simulink model "diophantineMPCSimulink"  (R2023b)
settings: Solver=VariableStepAuto  StartTime=0.0  StopTime=Tsim  RelTol=1e-3
undefined symbols (not defined in the file): denDelta, KF, KGp, Kr, numDelta, refFinalValue, refInitialValue, Tref, Ts
libraries: cstblocks x1
settings Model: Creator=klysm  LastModifiedBy=klysm

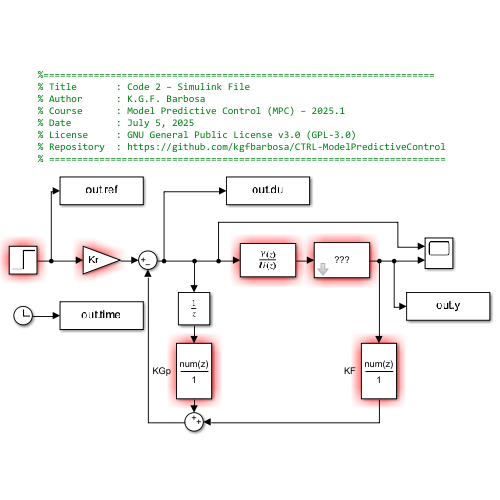
[thumbnail: Simulink's stored preview of the top-level diagram]
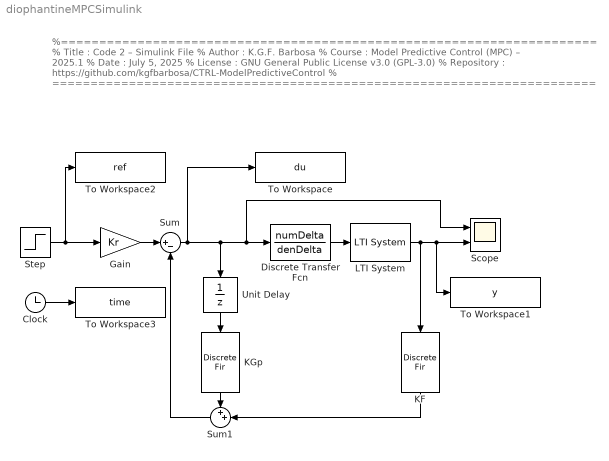
== system diophantineMPCSimulink ==
  note: %======================================================================
      | % Title : Code 2 – Simulink File
      | % Author : K.G.F. Barbosa
      | % Course : Model Predictive Control (MPC) – 2025.1
      | % Date : July 5, 2025
      | % License : GNU General Public License v3.0 (GPL-3.0)
      | % Repository : https://github.com/kgfbarbosa/CTRL-ModelPredictiveControl
      | % =======================================================================
  Clock : Clock
  Discrete Transfer Fcn : DiscreteTransferFcn  Numerator=numDelta  Denominator=denDelta
  Gain : Gain  Gain=Kr
  KF : DiscreteFir  Coefficients=KF
  KGp : DiscreteFir  Coefficients=KGp
  LTI System : cstblocks/LTI System  sys=Gz  IC=[]  PadeOrder=0
  Scope : Scope  NumInputPorts=2
  Step : Step  Time=Tref  Before=refInitialValue  After=refFinalValue  SampleTime=Ts
  Sum : Sum  Inputs=|+-
  Sum1 : Sum  Inputs=++|
  To Workspace : ToWorkspace  VariableName=du  SampleTime=Ts
      settings: Save2DSignal=2-D array (concatenate along first dimension)
  To Workspace1 : ToWorkspace  VariableName=y  SampleTime=Ts
      settings: Save2DSignal=2-D array (concatenate along first dimension)
  To Workspace2 : ToWorkspace  VariableName=ref  SampleTime=Ts
      settings: Save2DSignal=2-D array (concatenate along first dimension)
  To Workspace3 : ToWorkspace  VariableName=time  SampleTime=Ts
      settings: Save2DSignal=2-D array (concatenate along first dimension)
  Unit Delay : UnitDelay  SampleTime=Ts  HasFrameUpgradeWarning=on
  wires:
  LTI System/1 -> To Workspace1/1, Scope/2, KF/1
  Sum1/1 -> Sum/2
  Step/1 -> To Workspace2/1, Gain/1
  KGp/1 -> Sum1/1
  Discrete Transfer Fcn/1 -> LTI System/1
  KF/1 -> Sum1/2
  Unit Delay/1 -> KGp/1
  Sum/1 -> To Workspace/1, Discrete Transfer Fcn/1, Scope/1, Unit Delay/1
  Gain/1 -> Sum/1
  Clock/1 -> To Workspace3/1
